simulink model "Latest_Greatest"  (Simulink 10.1)
settings: Solver=ode4  StartTime=0  StopTime=15  FixedStep=DeltaT  RelTol=1e-3  EnableMultiTasking=on
InitFcn:
  | % Bifocal Relay Mirror Spacecraft (prior to payload installation) Dynamics Simulation          TA Sands
  | clear all;close all;clc;warning off all;
  | 
  | % Simulation run parameters
  | Rate=1000;  DeltaT=1/Rate;
  | 
  | % Maneuver Parameters
  | roll=0;  pitch=0; yaw=60;   roll=roll*pi/180; pitch=pitch*pi/180; yaw=yaw*pi/180;
  | SlewTime=5;   SACengage=0;
  | 
  | %Constants0
  | Re=6371.2e3;mu=398601.2e9;          %earth radius and universal gravitation constant
  | 
  | %Spacecraft orbit
  | h=0;                                     %orbit altitude
  | R=Re+h;                             %orbit radius from center of earth
  | we=0.000072921158553;   %earth's angular velocity rad/solar sec(Vallado)
  | wo=sqrt(mu/(Re+h)^3);        %orbit angular velocity
  | incln=36.6001*pi/180;          %Inclination assumed Monterey Latitude
  | epsilon=12*pi/180;  alphao=0;
  | uo=0; nuo=0;                        %Start S/C beneath subsolar point
  | beta=60; gamma=1.5;
  | a=0.545491852; b=0.314939867;  c=0.704226952;   %Assumed spacecraft rectangular size
  | Area=[b*c a*c a*b];                 %projected area~m^2 in body x,y,z directions
  | density=4.39e-14;
  | kpre=-9.9639/24/3600/180*pi*0;      %nodal precession constant assumed zero here
  | wn=kpre*(Re/(Re+h))^3.5*cos(incln); %nodal precession (zero eccentricity)
  | V=wo*(Re+h);
  | rho=asin(Re/(h+Re));                %earth angular radius
  | Cd=2.5;     psun=4.5E-6;            %Drag coefficient and solar pressure constant~N/m^2
  | Kaero=-0.5*Cd*V^2;   Psolar=2*psun;  %constants for aero and solar torque calculation
  | dL=[0.002 0.002 0.008];             %predicted distance between cp and cg
  | Kme=2.3390e-005;
  | 
  | %Spacecraft Magnetic Properties (assumed)
  | mresid=[0 0 0.01];                  %Spacecraft residual magnetic moment
  | M=mresid;                           %Magnetic unit dipole vector
  | K=7.943e15;
  | 
  | % ACTUAL Spacecraft Inertia conditions
  | Ix=90;   Iy=100;   Iz=250 ;
  | Ixy=-10;  Iyz=20;  Ixz=-10;
  | Imo=[Ix -Ixy -Ixz;
  |        -Ixy  Iy  -Iyz;
  |        -Ixz -Iyz  Iz];                  %Moment of inertia matrix
  | Iinv=inv(Imo);                      %Moment of inertia inverse goes in dynamics block
  | 
  | %Spacecraft initial Euler state angles and rates
  | phio=0;thetao=0;psio=0;                    %Initial Euler Angles
  | phidoto=0;thetadoto=0;psidoto=0;     %Initial Euler Rates
  | 
  | %Calculation of initial quaternion (qo) and angular momentum (Ho)
  | s1=sin(phio/2);s2=sin(thetao/2);s3=sin(psio/2);c1=cos(phio/2);c2=cos(thetao/2);c3=cos(psio/2);
  | q1o=s1*c2*c3-c1*s2*s3;
  | q2o=c1*s2*c3+s1*c2*s3;              %Wie pg. 321
  | q3o=c1*c2*s3-s1*s2*c3;
  | q4o=c1*c2*c3+s1*s2*s3;
  | S1=sin(phio);S2=sin(thetao);S3=sin(psio);C1=cos(phio);C2=cos(thetao);C3=cos(psio);
  | wxo=phidoto-psidoto*S2-wo*S3*C2;
  | wyo=thetadoto*C1+psidoto*C2*S1-wo*(C3*C1+S3*S2*S1);
  | ... (+55 lines)
StopFcn:
  | if flag==0; Hcmg=Hcmg;else;Hcmg=HcmgMP;end;
  | Hxcmg=[];Hycmg=[];Hzcmg=[];CondA=[]; CondA_MP=[];t=[]; SingPt=[];DetA=[];
  | for i=1:max(size(A));  t=[t i*DeltaT];  H=Hcmg(:,:,i); Hx=H(1,:);  Hy=H(2,:);  Hz=H(3,:);
  | detA=det(A(:,1:3,i));Hxcmg=[Hxcmg Hx];  Hycmg=[Hycmg Hy];  Hzcmg=[Hzcmg Hz];
  | CONDA=cond(A(:,:,i));
  | DetA=[DetA detA]; DetA=1./DetA;
  | CondA=[CondA CONDA];end;   %CondA=CondA./max(CondA); DetA=DetA./max(DetA);
  | Hmag=sqrt(Hxcmg.^2+Hycmg.^2+Hzcmg.^2);x=(max(t)-DeltaT);
  | 
  | InvCondA;
  | 
  | if flag==0; MaxInvCond=min(1./CondA(10*Rate+1:end));DELTA=delta;DELTAdot=deltadot;
  | else; MaxInvCond=min(1./CondA_MP(10*Rate+1:end));DELTA=delta_MP;DELTAdot=deltadot_MP;Hcmg=HcmgMP;end;
  | 
  | ERROR=(trajectory*180/pi-Euler);
  | 
  | figure(1); wdotTrajectory=[CMDTrajectory(:,1) CMDTrajectory(:,2) CMDTrajectory(:,3)];  wTrajectory=[CMDTrajectory(:,4) CMDTrajectory(:,5) CMDTrajectory(:,6)]; ThetaTrajectory=180/pi.*[trajectory(:,1) trajectory(:,2) trajectory(:,3)];
  | subplot(3,1,1); plot(t,wdotTrajectory,'linewidth',2); axis tight; grid; ylabel('\omega^d^o^t_C_M_D (deg)','fontsize',16); title('Desired Angle, Rate, Acceleration Trajectories','fontsize',16);   set(gca,'XTick',0:2:15);     set(gca,'XTickLabel',{' ',' ',' ',' ',' ',' ',' ',' ','15'});
  | subplot(3,1,2); plot(t,wTrajectory,'linewidth',2); axis tight; grid; ylabel('\omega_C_M_D (deg)','fontsize',16);set(gca,'XTick',0:2:15);     set(gca,'XTickLabel',{' ',' ',' ',' ',' ',' ',' ',' ','15'});
  | subplot(3,1,3); plot(t,ThetaTrajectory,'linewidth',2); axis tight; grid; ylabel('\theta_C_M_D (deg)','fontsize',16); xlabel('time (sec)','fontsize',16);
  | 
  | figure(2);
  | subplot(2,1,1);plot(t,Hmag,'LineWidth',3);   ylabel('|H_c_m_g|','Fontsize',16);grid;axis([0,x,0,3]); set(gca,'fontsize',16);set(gca,'XTickLabel',{' ',' ',' ',' ',' ',' ',' ',' ','15'});
  | subplot(2,1,2);plot(t,InvCondA,'linewidth',3);grid;xlabel('t(sec)','fontsize',14,'fontname','times');ylabel('Cond[A]','fontsize',14,'fontname','times');axis([0,max(t),0,21.82]); set(gca,'fontsize',16);
  | 
  | DELTA1=DELTA(1,:);DELTA2=DELTA(2,:);DELTA3=DELTA(3,:);DELTA4=DELTA(4,:);
  | DELTAdot1=DELTAdot(1,:);DELTAdot2=DELTAdot(2,:);DELTAdot3=DELTAdot(3,:);DELTAdot4=DELTAdot(4,:);
  | 
  | figure(3);subplot(4,1,1);plot(t,DELTA1,'LineWidth',3); title('Gimbal Angles','fontsize',16);ylabel('\theta_1(deg)','Fontsize',14);grid;axis tight; set(gca,'XTickLabel',{' ',' ',' ',' ',' ',' ',' ',' ','15'});set(gca,'fontsize',16);
  | subplot(4,1,2);plot(t,DELTA2,'LineWidth',3); ylabel('\theta_2(deg)','Fontsize',16);grid;axis tight; set(gca,'XTickLabel',{' ',' ',' ',' ',' ',' ',' ',' ','15'});set(gca,'fontsize',16);
  | subplot(4,1,3);plot(t,DELTA3,'LineWidth',3); ylabel('\theta_3(deg)','Fontsize',16);grid;axis tight; set(gca,'XTickLabel',{' ',' ',' ',' ',' ',' ',' ',' ','15'});set(gca,'fontsize',16);
  | subplot(4,1,4);plot(t,InvCondA,'linewidth',3);grid;xlabel('t(sec)','fontsize',14,'fontname','times');ylabel('Cond[A]','fontsize',14,'fontname','times');axis([0,max(t),0,21.82]); set(gca,'fontsize',16);
  | 
  | figure(4);subplot(4,1,1);plot(t,DELTAdot1,'LineWidth',3);  title('Gimbal Angle RATES','fontsize',16); ylabel('\theta_d_o_t_1(rad/s)','Fontsize',16);grid; axis([0,x,-pi*1.1,pi*1.1]);   set(gca,'XTickLabel',{' ',' ',' ',' ',' ',' ',' ',' ','15'});set(gca,'fontsize',16);
  | subplot(4,1,2);plot(t,DELTAdot2,'LineWidth',3);   ylabel('\theta_d_o_t_2(rad/s)','Fontsize',16);grid;axis([0,x,-pi*1.1,pi*1.1]);   set(gca,'XTickLabel',{' ',' ',' ',' ',' ',' ',' ',' ','15'});   set(gca,'fontsize',16);
  | subplot(4,1,3);plot(t,DELTAdot3,'LineWidth',3);   ylabel('\theta_d_o_t_3(rad/s)','Fontsize',16);grid;axis([0,x,-pi*1.1,pi*1.1]); set(gca,'XTickLabel',{' ',' ',' ',' ',' ',' ',' ',' ','15'});set(gca,'fontsize',16);
  | subplot(4,1,4);plot(t,InvCondA,'linewidth',3);grid;xlabel('t(sec)','fontsize',14,'fontname','times');ylabel('Cond[A]','fontsize',14,'fontname','times');axis([0,max(t),0,21.82]); set(gca,'fontsize',16);
  | 
  | figure(5);
  | subplot(4,1,1);plot(t,Hxcmg,'linewidth',3);axis([0,x,-3.25,3.25]);grid;ylabel('h_x/|h|','fontsize',16);title('Normalized Momentum','fontsize',16);set(gca,'XTickLabel',{' ',' ',' ',' ',' ',' ',' ',' ','15'});set(gca,'fontsize',16);
  | subplot(4,1,2);plot(t,Hycmg,'linewidth',3);axis([0,x,-3.25,3.25]);grid;ylabel('h_y/|h|','fontsize',16);set(gca,'XTickLabel',{' ',' ',' ',' ',' ',' ',' ',' ','15'});set(gca,'fontsize',16);
  | subplot(4,1,3);plot(t,Hzcmg,'linewidth',3);axis([0,x,-3.25,3.25]);grid;ylabel('h_z/|h|','fontsize',16);  set(gca,'XTickLabel',{' ',' ',' ',' ',' ',' ',' ',' ','15'});set(gca,'fontsize',16);
  | subplot(4,1,4);plot(t,InvCondA,'linewidth',3);grid;xlabel('t(sec)','fontsize',14,'fontname','times');ylabel('Cond[A]','fontsize',14,'fontname','times');axis([0,max(t),0,21.82]); set(gca,'fontsize',16);
  | 
  | figure(6); EulerX=Euler(:,1);EulerY=Euler(:,2);EulerZ=Euler(:,3);
  | subplot(4,1,1);plot(t,EulerX,'linewidth',3); axis([0,x,min(EulerX)*5,max(EulerX)*5]);grid;ylabel('\phi(deg)','fontsize',16);title('True Euler Angles','fontsize',14);  set(gca,'XTickLabel',{' ',' ',' ',' ',' ',' ',' ',' ','15'});  set(gca,'fontsize',16);
  | subplot(4,1,2);plot(t,EulerY,'linewidth',3);  axis([0,x,min(EulerY)*5,max(EulerY)*5]); grid;ylabel('\theta(deg)','fontsize',14);  set(gca,'XTickLabel',{' ',' ',' ',' ',' ',' ',' ',' ','15'}); set(gca,'fontsize',16);
  | subplot(4,1,3);plot(t,EulerZ,'linewidth',3);axis([0,x,min(EulerZ)*1.25,max(EulerZ)*1.25]);grid;  ylabel('\psi(deg)','fontsize',14);  set(gca,'XTickLabel',{' ',' ',' ',' ',' ',' ',' ',' ','15'});  set(gca,'fontsize',16);
  | subplot(4,1,4);plot(t,InvCondA,'linewidth',3);grid;xlabel('t(sec)','fontsize',14,'fontname','times');ylabel('Cond[A]','fontsize',14,'fontname','times');axis([0,max(t),0,21.82]); set(gca,'fontsize',16);
  | 
  | EX=ERROR(:,1);  EY=ERROR(:,2);     EZ=ERROR(:,3);
  | MeanXerror=mean(EX); Xmean=num2str(MeanXerror); xmean=['\mu_\phi=', Xmean];
  | STDx=std(EX);Xsigma=num2str(STDx);SigmaX=['    \sigma_x=' Xsigma];  xlegend=[xmean, SigmaX];
  | MeanYerror=mean(EY); Ymean=num2str(MeanYerror); ymean=['\mu_\theta=', Ymean];
  | STDy=std(EY); Ysigma=num2str(STDy);SigmaY=['    \sigma_y=' Ysigma]; ylegend=[ymean, SigmaY];
  | MeanZerror=mean(EZ); Zmean=num2str(MeanZerror); zmean=['\mu_\psi=', Zmean];
  | STDz=std(EZ);Zsigma=num2str(STDz);SigmaZ=['    \sigma_z=' Zsigma]; zlegend=[zmean, SigmaZ];
  | MeanError=[MeanXerror MeanYerror MeanZerror];  StdDev=[STDx STDy STDz];
  | 
  | figure(7);
  | ... (+78 lines)
undefined symbols (not defined in the file): magnitude, svd
libraries: aerospace x3, simulink_need_slupdate x2, dspadpt3 x2, dspinverses x1
(part 2 of 2)

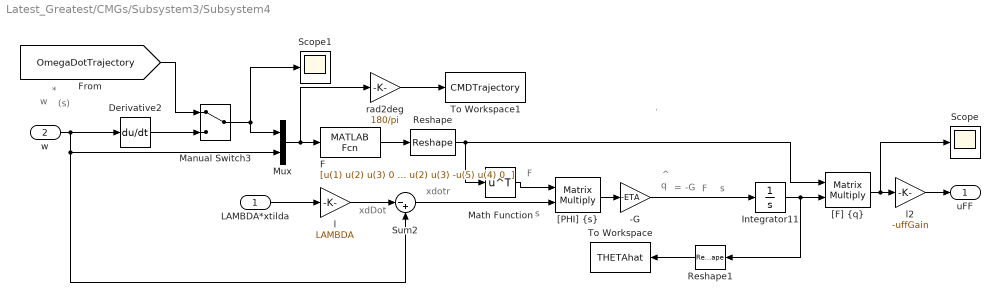
== system Latest_Greatest/CMGs/Subsystem3/Subsystem4 ==
  note: xdotr
  note: s
  note: xdDot
  note: F
  note: -G
  note: F
  note: s
  note: =
  note: .
  note: ^
  note: q
  note: *
  note: (s)
  note: w
  LAMBDA*xtilda : Inport
  w : Inport  Port=2
  -G : Gain  Gain=-ETA  SaturateOnIntegerOverflow=on  OutDataTypeStr=Inherit: Same as input  ParamDataTypeStr=Inherit: Same as input
  Derivative2 : Derivative
  F : MATLABFcn  MATLABFcn="[u(1) u(2) u(3) 0 0 0 0 -u(6) u(5);  0 u(1) 0 u(2) u(3) 0 u(6) 0 u(4);  0 0 u(1) 0 u(2) u(3) -u(5) u(4) 0  ]"
  Integrator11 : Integrator  InitialCondition=THETAo
  Manual Switch3 : ManualSwitch
  Math Function : Math  Operator=transpose  SignedPower=on  SaturateOnIntegerOverflow=on
  Mux : Mux  Inputs=2
  Reshape : Reshape  OutputDimensionality=Customize  OutputDimensions=[3,9]
  Reshape1 : Reshape  OutputDimensions=[1,9]
  Scope : Scope
  Scope1 : Scope
  Sum2 : Sum  Inputs=|-+  SaturateOnIntegerOverflow=on
  To Workspace : ToWorkspace  VariableName=THETAhat  SampleTime=-1
  To Workspace1 : ToWorkspace  VariableName=CMDTrajectory  SampleTime=-1
  "[F] {q}" : Product  Multiplication=Matrix(*)  SaturateOnIntegerOverflow=on  OutDataTypeStr=Inherit: Same as first input
  "[PHI] {s}" : Product  Multiplication=Matrix(*)  SaturateOnIntegerOverflow=on  OutDataTypeStr=Inherit: Same as first input
  l : Gain  Gain=LAMBDA  SaturateOnIntegerOverflow=on  OutDataTypeStr=Inherit: Same as input  ParamDataTypeStr=Inherit: Same as input
  l2 : Gain  Gain=-uffGain  SaturateOnIntegerOverflow=on  OutDataTypeStr=Inherit: Same as input  ParamDataTypeStr=Inherit: Same as input
  rad2deg : Gain  Gain=180/pi  SaturateOnIntegerOverflow=on  OutDataTypeStr=Inherit: Same as input  ParamDataTypeStr=Inherit: Same as input
  uFF : Outport  VectorParamsAs1DForOutWhenUnconnected=off
  wires:
  LAMBDA*xtilda/1 -> l/1
  l/1 -> Sum2/1
  Sum2/1 -> "[PHI] {s}"/2
  "[PHI] {s}"/1 -> -G/1
  F/1 -> Reshape/1
  w/1 -> Derivative2/1, Mux/2, Sum2/2
  Mux/1 -> F/1, rad2deg/1
  -G/1 -> Integrator11/1
  "[F] {q}"/1 -> l2/1, Scope/1
  Reshape/1 -> "[F] {q}"/1, Math Function/1
  Math Function/1 -> "[PHI] {s}"/1
  Reshape1/1 -> To Workspace/1
  Integrator11/1 -> "[F] {q}"/2, Reshape1/1
  rad2deg/1 -> To Workspace1/1
  l2/1 -> uFF/1
  Manual Switch3/1 -> Mux/1, Scope1/1
  [OmegaDotTrajectory] -> Manual Switch3/1
  Derivative2/1 -> Manual Switch3/2

== system Latest_Greatest/Subsystem2/Tgg/Select ci3 ==
  U : Inport
  C11 : Fcn  Expr=u[3]
  C12 : Fcn  Expr=u[6]
  C13 : Fcn  Expr=u[9]
  Mux2 : Mux  Inputs=3
  U(E) : Outport  VectorParamsAs1DForOutWhenUnconnected=off
  wires:
  C11/1 -> Mux2/1
  C12/1 -> Mux2/2
  C13/1 -> Mux2/3
  U/1 -> C12/1, C11/1, C13/1
  Mux2/1 -> U(E)/1

== system Latest_Greatest/Subsystem3/Subsystem1/Euler Angle ==
  note: q
  note: f
  note: y
  note: q
  DCM : Inport
  -asin(C13) : Fcn  Expr=-asin(u[3])
  C12 : Fcn  Expr=u[2]
  C23 : Fcn  Expr=u[6]
  Fcn : Fcn  Expr="asin(u[2]/cos(u[1])  )"
  Fcn1 : Fcn  Expr=asin(u[1]/cos(u[2]))
  Mux : Mux  Inputs=3
  Mux1 : Mux  Inputs=2
  Mux2 : Mux  Inputs=2
  Euler Angles : Outport  VectorParamsAs1DForOutWhenUnconnected=off
  wires:
  C12/1 -> Mux2/2
  Fcn/1 -> Mux/3
  Mux2/1 -> Fcn/1
  C23/1 -> Mux1/1
  -asin(C13)/1 -> Mux2/1, Mux1/2, Mux/2
  Fcn1/1 -> Mux/1
  Mux1/1 -> Fcn1/1
  DCM/1 -> C12/1, C23/1, -asin(C13)/1
  Mux/1 -> Euler Angles/1

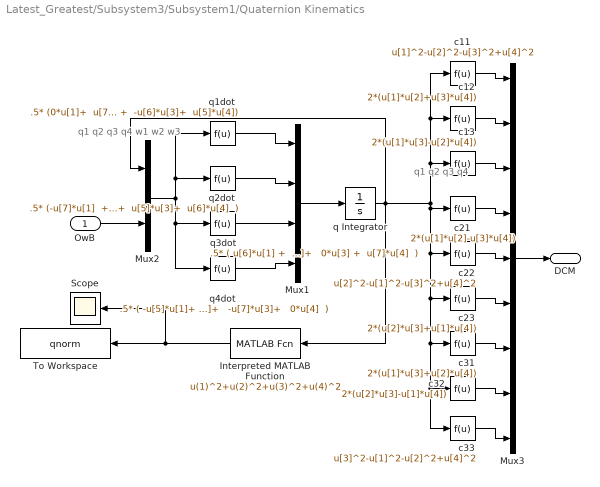
== system Latest_Greatest/Subsystem3/Subsystem1/Quaternion Kinematics ==
  note: q1
      | q2
      | q3
      | q4
      | w1
      | w2
      | w3
  note: q1
      | q2
      | q3
      | q4
  OwB : Inport
  Interpreted MATLAB Function : MATLABFcn  MATLABFcn=u(1)^2+u(2)^2+u(3)^2+u(4)^2
  Mux1 : Mux
  Mux2 : Mux  Inputs=2
  Mux3 : Mux  Inputs=9
  Scope : Scope
  To Workspace : ToWorkspace  VariableName=qnorm  SampleTime=-1
  c11 : Fcn  Expr=u[1]^2-u[2]^2-u[3]^2+u[4]^2
  c12 : Fcn  Expr=2*(u[1]*u[2]+u[3]*u[4])
  c13 : Fcn  Expr=2*(u[1]*u[3]-u[2]*u[4])
  c21 : Fcn  Expr=2*(u[1]*u[2]-u[3]*u[4])
  c22 : Fcn  Expr=u[2]^2-u[1]^2-u[3]^2+u[4]^2
  c23 : Fcn  Expr=2*(u[2]*u[3]+u[1]*u[4])
  c31 : Fcn  Expr=2*(u[1]*u[3]+u[2]*u[4])
  c32 : Fcn  Expr=2*(u[2]*u[3]-u[1]*u[4])
  c33 : Fcn  Expr=u[3]^2-u[1]^2-u[2]^2+u[4]^2
  q Integrator : Integrator  InitialCondition=qo
  q1dot : Fcn  Expr=".5* (0*u[1]+  u[7]*u[2] +  -u[6]*u[3]+  u[5]*u[4])"
  q2dot : Fcn  Expr=".5* (-u[7]*u[1]  +  0*u[2]+  u[5]*u[3]+  u[6]*u[4]  )"
  q3dot : Fcn  Expr=".5* ( u[6]*u[1] +  -u[5]*u[2]+   0*u[3] +  u[7]*u[4]  )"
  q4dot : Fcn  Expr=".5* ( -u[5]*u[1]+   -u[6]*u[2]+   -u[7]*u[3]+   0*u[4]  )"
  DCM : Outport  VectorParamsAs1DForOutWhenUnconnected=off
  wires:
  OwB/1 -> Mux2/2
  q1dot/1 -> Mux1/1
  q2dot/1 -> Mux1/2
  q3dot/1 -> Mux1/3
  q4dot/1 -> Mux1/4
  Mux1/1 -> q Integrator/1
  q Integrator/1 -> Interpreted MATLAB Function/1, c12/1, c11/1, c13/1, c21/1, c22/1, c23/1, c31/1, c33/1, c32/1, Mux2/1
  c11/1 -> Mux3/1
  c12/1 -> Mux3/2
  c13/1 -> Mux3/3
  c22/1 -> Mux3/5
  c21/1 -> Mux3/4
  c23/1 -> Mux3/6
  c31/1 -> Mux3/7
  c32/1 -> Mux3/8
  c33/1 -> Mux3/9
  Mux3/1 -> DCM/1
  Mux2/1 -> q2dot/1, q1dot/1, q3dot/1, q4dot/1
  Interpreted MATLAB Function/1 -> To Workspace/1, Scope/1

== system Latest_Greatest/Subsystem3/Subsystem1/Select ci2 ==
  U : Inport
  C12 : Fcn  Expr=u[2]
  C22 : Fcn  Expr=u[5]
  C32 : Fcn  Expr=u[8]
  Mux2 : Mux  Inputs=3
  U(E) : Outport  VectorParamsAs1DForOutWhenUnconnected=off
  wires:
  C12/1 -> Mux2/1
  C22/1 -> Mux2/2
  C32/1 -> Mux2/3
  U/1 -> C32/1, C22/1, C12/1
  Mux2/1 -> U(E)/1

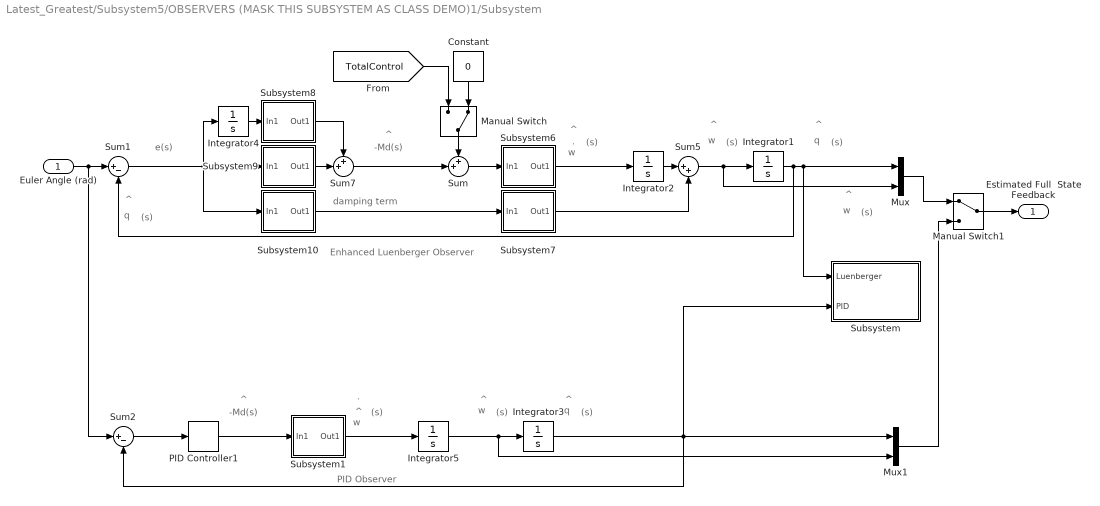
== system Latest_Greatest/Subsystem5/OBSERVERS (MASK THIS SUBSYSTEM AS CLASS DEMO)1/Subsystem ==
  note: PID Observer
  note: -Md(s)
  note: ^
  note: ^
  note: (s)
  note: w
  note: (s)
  note: .
  note: ^
  note: w
  note: e(s)
  note: q
  note: ^
  note: (s)
  note: ^
  note: (s)
  note: w
  note: damping term
  note: Enhanced Luenberger Observer
  note: ^
  note: (s)
  note: w
  note: (s)
  note: .
  note: ^
  note: w
  note: (s)
  note: ^
  note: q
  note: ^
  note: -Md(s)
  note: (s)
  note: ^
  note: q
  Euler Angle (rad) : Inport
  Constant : Constant  Value=0
  Integrator{1..5} (5 alike) : Integrator
  Manual Switch : ManualSwitch  CurrentSetting=0
  Manual Switch1 : ManualSwitch
  Mux : Mux  Inputs=2
  Mux1 : Mux  Inputs=2
  PID Controller1 : simulink_need_slupdate/PID Controller  P=Kpo  I=Kio  D=Kdo
  Subsystem : Subsystem
      mask Display: disp('Scopes')
  Subsystem1 : Subsystem
      mask Display: disp('1/J^p')
  Subsystem10 : Subsystem
      mask Display: disp('Kdo')
  Subsystem6 : Subsystem
      mask Display: disp('1/J^p')
  Subsystem7 : Subsystem
      mask Display: disp('1/J^p')
  Subsystem8 : Subsystem
      mask Display: disp('Kio')
  Subsystem9 : Subsystem
      mask Display: disp('Kpo')
  Sum : Sum  Inputs=++|
  Sum1 : Sum  Inputs=|+-
  Sum2 : Sum  Inputs=|+-
  Sum5 : Sum  Inputs=|++
  Sum7 : Sum  Inputs=++|
  Estimated Full  State Feedback : Outport  VectorParamsAs1DForOutWhenUnconnected=off
  wires:
  Manual Switch1/1 -> Estimated Full  State Feedback/1
  Mux1/1 -> Manual Switch1/2
  Mux/1 -> Manual Switch1/1
  PID Controller1/1 -> Subsystem1/1(In1)
  Integrator3/1 -> Mux1/1, Subsystem/2(PID), Sum2/2
  Integrator5/1 -> Mux1/2, Integrator3/1
  Subsystem1/1(Out1) -> Integrator5/1
  Manual Switch/1 -> Sum/1
  Constant/1 -> Manual Switch/2
  [TotalControl] -> Manual Switch/1
  Euler Angle (rad)/1 -> Sum1/1, Sum2/1
  Sum1/1 -> Subsystem10/1(In1), Subsystem9/1(In1), Integrator4/1
  Sum/1 -> Subsystem6/1(In1)
  Sum7/1 -> Sum/2
  Integrator1/1 -> Subsystem/1(Luenberger), Mux/1, Sum1/2
  Sum5/1 -> Mux/2, Integrator1/1
  Integrator4/1 -> Subsystem8/1(In1)
  Subsystem10/1(Out1) -> Subsystem7/1(In1)
  Subsystem9/1(Out1) -> Sum7/2
  Subsystem8/1(Out1) -> Sum7/1
  Subsystem7/1(Out1) -> Sum5/2
  Integrator2/1 -> Sum5/1
  Subsystem6/1(Out1) -> Integrator2/1
  Sum2/1 -> PID Controller1/1

== system Latest_Greatest/CMGs/Subsystem3/Subsystem1/Subsystem25 ==
  In1 : Inport
  Clock : Clock
  Ki : Gain  Gain=-Ki
  To Workspace : ToWorkspace  VariableName=t  SampleTime=-1
  Out1 : Outport  VectorParamsAs1DForOutWhenUnconnected=off
  wires:
  Clock/1 -> To Workspace/1
  In1/1 -> Ki/1
  Ki/1 -> Out1/1

== system Latest_Greatest/CMGs/Subsystem3/Subsystem1/Subsystem26 ==
  In1 : Inport
  Gain : Gain  Gain=-Kp
  Out1 : Outport  VectorParamsAs1DForOutWhenUnconnected=off
  wires:
  Gain/1 -> Out1/1
  In1/1 -> Gain/1

== system Latest_Greatest/CMGs/Subsystem3/Subsystem1/Subsystem27 ==
  In1 : Inport
  Gain : Gain  Gain=-Kd
  Out1 : Outport  VectorParamsAs1DForOutWhenUnconnected=off
  wires:
  In1/1 -> Gain/1
  Gain/1 -> Out1/1

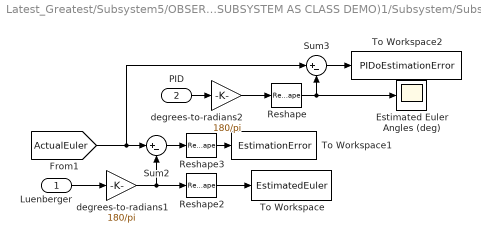
== system Latest_Greatest/Subsystem5/OBSERVERS (MASK THIS SUBSYSTEM AS CLASS DEMO)1/Subsystem/Subsystem ==
  Luenberger : Inport
  PID : Inport  Port=2
  Estimated Euler Angles (deg) : Scope
      settings: StopFcn=|
      | %Simulink figure properties
      | shh=get(0,'ShowHiddenHandles');
      | set(0,'ShowHiddenHandles','On')
      | set(gcf,'menubar','figure')
      | set(gcf,'CloseRequestFcn','closereq')
      | set(gcf,'DefaultLineClipping','Off')
      | set(0,'ShowHiddenHandles',shh)
  Reshape : Reshape
  Reshape2 : Reshape  OutputDimensions=[1,9]
  Reshape3 : Reshape  OutputDimensions=[1,9]
  Sum2 : Sum  Inputs=|+-
  Sum3 : Sum  Inputs=|+-
  To Workspace : ToWorkspace  VariableName=EstimatedEuler  SampleTime=-1
  To Workspace1 : ToWorkspace  VariableName=EstimationError  SampleTime=-1
  To Workspace2 : ToWorkspace  VariableName=PIDoEstimationError  SampleTime=-1
  degrees-to-radians1 : Gain  Gain=180/pi
  degrees-to-radians2 : Gain  Gain=180/pi
  wires:
  degrees-to-radians2/1 -> Reshape/1
  Reshape/1 -> Estimated Euler Angles (deg)/1, Sum3/2
  PID/1 -> degrees-to-radians2/1
  Sum3/1 -> To Workspace2/1
  Luenberger/1 -> degrees-to-radians1/1
  Reshape3/1 -> To Workspace1/1
  Reshape2/1 -> To Workspace/1
  [ActualEuler] -> Sum3/1, Sum2/1
  Sum2/1 -> Reshape3/1
  degrees-to-radians1/1 -> Reshape2/1, Sum2/2

== system Latest_Greatest/Subsystem5/OBSERVERS (MASK THIS SUBSYSTEM AS CLASS DEMO)1/Subsystem/Subsystem1 ==
  In1 : Inport
  Gain : Gain  Gain=Iinv  Multiplication=Matrix(K*u)
  Out1 : Outport  VectorParamsAs1DForOutWhenUnconnected=off
  wires:
  In1/1 -> Gain/1
  Gain/1 -> Out1/1

== system Latest_Greatest/Subsystem5/OBSERVERS (MASK THIS SUBSYSTEM AS CLASS DEMO)1/Subsystem/Subsystem10 ==
  In1 : Inport
  Gain : Gain  Gain=Kdo
  Out1 : Outport  VectorParamsAs1DForOutWhenUnconnected=off
  wires:
  Gain/1 -> Out1/1
  In1/1 -> Gain/1

== system Latest_Greatest/Subsystem5/OBSERVERS (MASK THIS SUBSYSTEM AS CLASS DEMO)1/Subsystem/Subsystem6 ==
  In1 : Inport
  Gain : Gain  Gain=Iinv  Multiplication=Matrix(K*u)
  Out1 : Outport  VectorParamsAs1DForOutWhenUnconnected=off
  wires:
  Gain/1 -> Out1/1
  In1/1 -> Gain/1

== system Latest_Greatest/Subsystem5/OBSERVERS (MASK THIS SUBSYSTEM AS CLASS DEMO)1/Subsystem/Subsystem7 ==
  In1 : Inport
  Gain : Gain  Gain=Iinv  Multiplication=Matrix(K*u)
  Out1 : Outport  VectorParamsAs1DForOutWhenUnconnected=off
  wires:
  In1/1 -> Gain/1
  Gain/1 -> Out1/1

== system Latest_Greatest/Subsystem5/OBSERVERS (MASK THIS SUBSYSTEM AS CLASS DEMO)1/Subsystem/Subsystem8 ==
  In1 : Inport
  Gain : Gain  Gain=Kio
  Out1 : Outport  VectorParamsAs1DForOutWhenUnconnected=off
  wires:
  Gain/1 -> Out1/1
  In1/1 -> Gain/1

== system Latest_Greatest/Subsystem5/OBSERVERS (MASK THIS SUBSYSTEM AS CLASS DEMO)1/Subsystem/Subsystem9 ==
  In1 : Inport
  Gain : Gain  Gain=Kpo
  Out1 : Outport  VectorParamsAs1DForOutWhenUnconnected=off
  wires:
  In1/1 -> Gain/1
  Gain/1 -> Out1/1
